simulink model "FlexSensor_2in2_v2"  (R2017b)
settings: Solver=VariableStepAuto  StartTime=0.0  StopTime=inf  RelTol=1e-3
libraries: fl_lib x16, nesl_utility x10
settings Model: Creator=stark  LastModifiedBy=stark

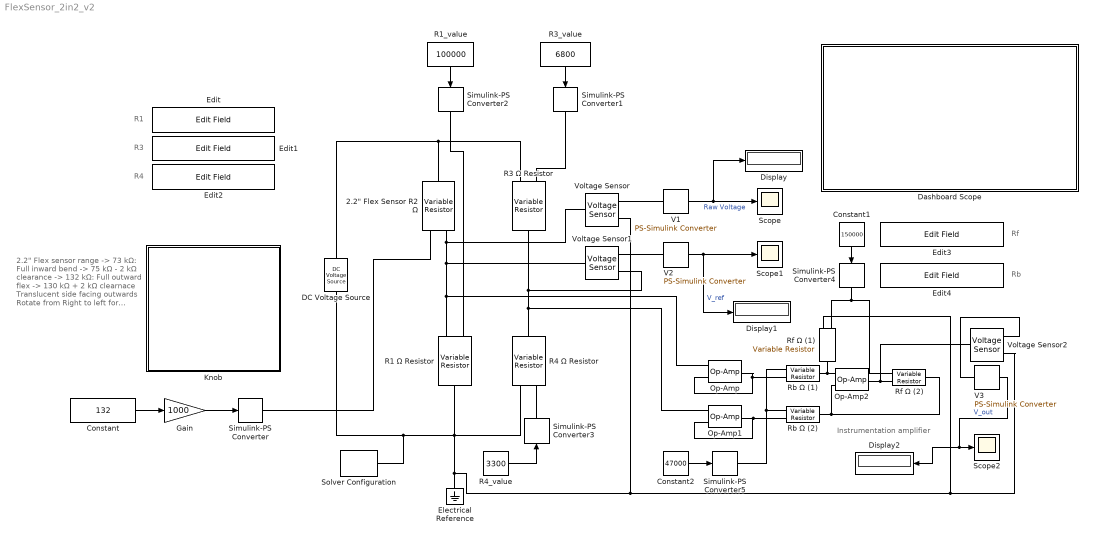
== system FlexSensor_2in2_v2 ==
  note: Rf
  note: Instrumentation amplifier
  note: R4
  note: R1
  note: 2.2" Flex sensor range
      | -> 73 kΩ: Full inward bend
      | -> 75 kΩ - 2 kΩ clearance
      | -> 132 kΩ: Full outward flex
      | -> 130 kΩ + 2 kΩ clearnace
      | Translucent side facing outwards
      | Rotate from Right to left for
      | clentching inwards and Left
      | to right for opening outwards
  note: R3
  note: Rb
  "2.2\" Flex Sensor R2 Ω" : fl_lib/Electrical/Electrical Elements/Variable Resistor  Rmin=0 Ohm  i_specify=off  i_priority=None  i=0 A  i_nominal_specify=off  i_nominal_unit=A  i_nominal_value=1  v_specify=off  v_priority=None  v=0 V  v_nominal_specify=off  v_nominal_unit=V  v_nominal_value=1
  Constant : Constant  Value=132  OutMin=[73]  OutMax=[132]
  Constant1 : Constant  Value=150000
  Constant2 : Constant  Value=47000
  DC Voltage Source : fl_lib/Electrical/Electrical Sources/DC Voltage Source  v0=5 V
  Dashboard Scope : Subsystem  DialogController=hmiCreateDDGDialog  IsWebBlock=on  mask(MWDashboardBlock){webBlockId=80df2397-1243-4d8f-ab33-ab65e66ae50b, webBlockType=sdiscope, ShowInitialText=on, HMISrcModelName=FlexSensor_2in2_v2}
      mask prompts: webBlockId "WebBlock Id"; webBlockType "WebBlock Type"; HMISrcModelName "Source Model"
      mask help: SimulinkHMI:dialogs:HMIScopeDialogDesc
      mask Help: helpview([docroot '/mapfiles/simulink.map'], 'hmi_scope')
      mask Display:
      | if strcmp(get_param(bdroot(gcb),'BlockDiagramType'), 'library')
      |     image([(matlabroot) '/toolbox/simulink/hmi/icons/DashboardScope.png']);
      | end
  Display : Display
  Display1 : Display
  Display2 : Display
  Edit : EditField  WebBlockId=8  ModelName=FlexSensor_2in2_v2  LabelPosition=Hide  ShowInitialText=off  Alignment=Center
  Edit1 : EditField  WebBlockId=9  ModelName=FlexSensor_2in2_v2  LabelPosition=Hide  ShowInitialText=off  Alignment=Center
  Edit2 : EditField  WebBlockId=10  ModelName=FlexSensor_2in2_v2  LabelPosition=Hide  ShowInitialText=off  Alignment=Center
  Edit3 : EditField  WebBlockId=45  ModelName=FlexSensor_2in2_v2  LabelPosition=Hide  ShowInitialText=off  Alignment=Center
  Edit4 : EditField  WebBlockId=49  ModelName=FlexSensor_2in2_v2  LabelPosition=Hide  ShowInitialText=off  Alignment=Center
  Electrical Reference : fl_lib/Electrical/Electrical Elements/Electrical Reference
  Gain : Gain  Gain=1000
  Knob : Subsystem  DialogController=hmiCreateDDGDialog  IsWebBlock=on  mask(MWDashboardBlock){webBlockId=85848859-5c60-4759-b489-606f39201498, webBlockType=continuousknob, ShowInLibBrowser=on, ShowInitialText=on, HMISrcModelName=FlexSensor_2in2_v2}
      mask prompts: webBlockId "WebBlock Id"; webBlockType "WebBlock Type"; HMISrcModelName "Source Model"
      mask help: SimulinkHMI:dialogs:ContinuousKnobDialogDesc
      mask Help: helpview([docroot '/mapfiles/simulink.map'], 'hmi_knob')
      mask Display:
      | if strcmp(get_param(bdroot(gcb),'BlockDiagramType'), 'library')
      |     image([(matlabroot) '/toolbox/simulink/hmi/icons/ContinuousKnob.png']);
      | end
  Op-Amp : fl_lib/Electrical/Electrical Elements/Op-Amp  outI_specify=off  outI_priority=None  outI=0 A  outI_nominal_specify=off  outI_nominal_unit=A  outI_nominal_value=1
  Op-Amp1 : fl_lib/Electrical/Electrical Elements/Op-Amp  outI_specify=off  outI_priority=None  outI=0 A  outI_nominal_specify=off  outI_nominal_unit=A  outI_nominal_value=1
  Op-Amp2 : fl_lib/Electrical/Electrical Elements/Op-Amp  outI_specify=off  outI_priority=None  outI=0 A  outI_nominal_specify=off  outI_nominal_unit=A  outI_nominal_value=1
  R1 Ω Resistor : fl_lib/Electrical/Electrical Elements/Variable Resistor  Rmin=0 Ohm  i_specify=off  i_priority=None  i=0 A  i_nominal_specify=off  i_nominal_unit=A  i_nominal_value=1  v_specify=off  v_priority=None  v=0 V  v_nominal_specify=off  v_nominal_unit=V  v_nominal_value=1
  R1_value : Constant  Value=100000
  R3 Ω Resistor : fl_lib/Electrical/Electrical Elements/Variable Resistor  Rmin=0 Ohm  i_specify=off  i_priority=None  i=0 A  i_nominal_specify=off  i_nominal_unit=A  i_nominal_value=1  v_specify=off  v_priority=None  v=0 V  v_nominal_specify=off  v_nominal_unit=V  v_nominal_value=1
  R3_value : Constant  Value=6800
  R4 Ω Resistor : fl_lib/Electrical/Electrical Elements/Variable Resistor  Rmin=0 Ohm  i_specify=off  i_priority=None  i=0 A  i_nominal_specify=off  i_nominal_unit=A  i_nominal_value=1  v_specify=off  v_priority=None  v=0 V  v_nominal_specify=off  v_nominal_unit=V  v_nominal_value=1
  R4_value : Constant  Value=3300
  Rb Ω (1) : fl_lib/Electrical/Electrical Elements/Variable Resistor  Rmin=0 Ohm  i_specify=off  i_priority=None  i=0 A  i_nominal_specify=off  i_nominal_unit=A  i_nominal_value=1  v_specify=off  v_priority=None  v=0 V  v_nominal_specify=off  v_nominal_unit=V  v_nominal_value=1
  Rb Ω (2) : fl_lib/Electrical/Electrical Elements/Variable Resistor  Rmin=0 Ohm  i_specify=off  i_priority=None  i=0 A  i_nominal_specify=off  i_nominal_unit=A  i_nominal_value=1  v_specify=off  v_priority=None  v=0 V  v_nominal_specify=off  v_nominal_unit=V  v_nominal_value=1
  Rf Ω (1) : fl_lib/Electrical/Electrical Elements/Variable Resistor  Rmin=0 Ohm  i_specify=off  i_priority=None  i=0 A  i_nominal_specify=off  i_nominal_unit=A  i_nominal_value=1  v_specify=off  v_priority=None  v=0 V  v_nominal_specify=off  v_nominal_unit=V  v_nominal_value=1
  Rf Ω (2) : fl_lib/Electrical/Electrical Elements/Variable Resistor  Rmin=0 Ohm  i_specify=off  i_priority=None  i=0 A  i_nominal_specify=off  i_nominal_unit=A  i_nominal_value=1  v_specify=off  v_priority=None  v=0 V  v_nominal_specify=off  v_nominal_unit=V  v_nominal_value=1
  Scope : Scope
  Scope1 : Scope
  Scope2 : Scope
  Simulink-PS Converter{,1..5} (6 alike) : nesl_utility/Simulink-PS Converter  PhysicalDomain=network_engine_domain  SubClassName=ps_input  LeftPortType=input  RightPortType=output  PseudoPeriodic=off  Frequencies=[]  NoiseDistribution=none  NoiseParameters=[]  Unit=1  AffineConversion=off  FilteringAndDerivatives=provide  SimscapeFilterOrder=1  InputFilterTimeConstant=0.001  UdotUserProvided=0
  Solver Configuration : nesl_utility/Solver Configuration  PhysicalDomain=network_engine_domain  SubClassName=solver  LeftPortType=input  RightPortType=generic  Accelerate=off  Tones=[]  Harmonics=[]  SimulateNoise=off  Profile=off  UseLocalSampling=off  EnableSwitchedLinearOptims=on  FrequencyDomain=off  UseCCode=off  RelTol=0.001  AbsTol=1e-06  MinStep=1e-09  ToWorkspace=off  RevertToSquareIcSolve=off  NumHomotopyIterations=100  PhasorMode=off  PhasorModeNumHarmonics=1  DoDC=off  ResidualTolerance=1e-09  UseLocalSolver=off  LocalSolverChoice=NE_BACKWARD_EULER_ADVANCER  LocalSolverSampleTime=0.001  DoFixedCost=off  MaxNonlinIter=3  MaxModeIter=2  LinearAlgebra=Sparse  DelaysMemoryBudget=1024  AutomaticFiltering=on  FilteringTimeConstant=0.001
  V1 : nesl_utility/PS-Simulink Converter  PhysicalDomain=network_engine_domain  SubClassName=ps_output  LeftPortType=input  RightPortType=output  PseudoPeriodic=off  Frequencies=[]  Unit=1  AffineConversion=off
  V2 : nesl_utility/PS-Simulink Converter  PhysicalDomain=network_engine_domain  SubClassName=ps_output  LeftPortType=input  RightPortType=output  PseudoPeriodic=off  Frequencies=[]  Unit=1  AffineConversion=off
  V3 : nesl_utility/PS-Simulink Converter  PhysicalDomain=network_engine_domain  SubClassName=ps_output  LeftPortType=input  RightPortType=output  PseudoPeriodic=off  Frequencies=[]  Unit=1  AffineConversion=off
  Voltage Sensor : fl_lib/Electrical/Electrical Sensors/Voltage Sensor
  Voltage Sensor1 : fl_lib/Electrical/Electrical Sensors/Voltage Sensor
  Voltage Sensor2 : fl_lib/Electrical/Electrical Sensors/Voltage Sensor
  wires:
  Gain/1 -> Simulink-PS Converter/1
  V2/1 -> Display1/1, Scope1/1  "V_ref"
  R1_value/1 -> Simulink-PS Converter2/1
  R3_value/1 -> Simulink-PS Converter1/1
  R4_value/1 -> Simulink-PS Converter3/1
  V1/1 -> Display/1, Scope/1  "Raw Voltage"
  Constant/1 -> Gain/1
  Constant1/1 -> Simulink-PS Converter4/1
  Constant2/1 -> Simulink-PS Converter5/1
  V3/1 -> Display2/1, Scope2/1  "V_out"
  connections:
  Voltage Sensor1/LConn1 -- Op-Amp/LConn1 -- R1 Ω Resistor/LConn2 -- "2.2\" Flex Sensor R2 Ω"/LConn2 -- Voltage Sensor/LConn1
  R1 Ω Resistor/RConn1 -- DC Voltage Source/RConn1 -- Solver Configuration/RConn1 -- Voltage Sensor2/RConn2 -- Rf Ω (1)/LConn2 -- Voltage Sensor/RConn2 -- Electrical Reference/LConn1 -- R4 Ω Resistor/LConn2
  DC Voltage Source/LConn1 -- R3 Ω Resistor/LConn2 -- "2.2\" Flex Sensor R2 Ω"/RConn1
  R3 Ω Resistor/RConn1 -- Op-Amp1/LConn1 -- R4 Ω Resistor/RConn1 -- Voltage Sensor1/RConn2
  Simulink-PS Converter1/RConn1 -- R3 Ω Resistor/LConn1
  Simulink-PS Converter2/RConn1 -- R1 Ω Resistor/LConn1
  Simulink-PS Converter/RConn1 -- "2.2\" Flex Sensor R2 Ω"/LConn1
  V2/LConn1 -- Voltage Sensor1/RConn1
  V1/LConn1 -- Voltage Sensor/RConn1
  Simulink-PS Converter3/RConn1 -- R4 Ω Resistor/LConn1
  Op-Amp/RConn1 -- Rb Ω (1)/LConn2 -- Op-Amp/LConn2
  Op-Amp1/RConn1 -- Op-Amp1/LConn2 -- Rb Ω (2)/LConn2
  Rb Ω (1)/RConn1 -- Rf Ω (1)/RConn1 -- Op-Amp2/LConn1
  Rb Ω (2)/RConn1 -- Rf Ω (2)/RConn1 -- Op-Amp2/LConn2
  Rf Ω (2)/LConn2 -- Voltage Sensor2/LConn1 -- Op-Amp2/RConn1
  Simulink-PS Converter4/RConn1 -- Rf Ω (2)/LConn1 -- Rf Ω (1)/LConn1
  Simulink-PS Converter5/RConn1 -- Rb Ω (2)/LConn1 -- Rb Ω (1)/LConn1
  V3/LConn1 -- Voltage Sensor2/RConn1

== system FlexSensor_2in2_v2/Dashboard Scope ==

== system FlexSensor_2in2_v2/Knob ==
